simulink model "Ali_model"  (R2014b)
settings: Solver=ode4  StartTime=0.2  StopTime=11  FixedStep=0.001  RelTol=1e-3
libraries: simulink x1
settings Model: Creator=mshahria  LastModifiedBy=nlashkar

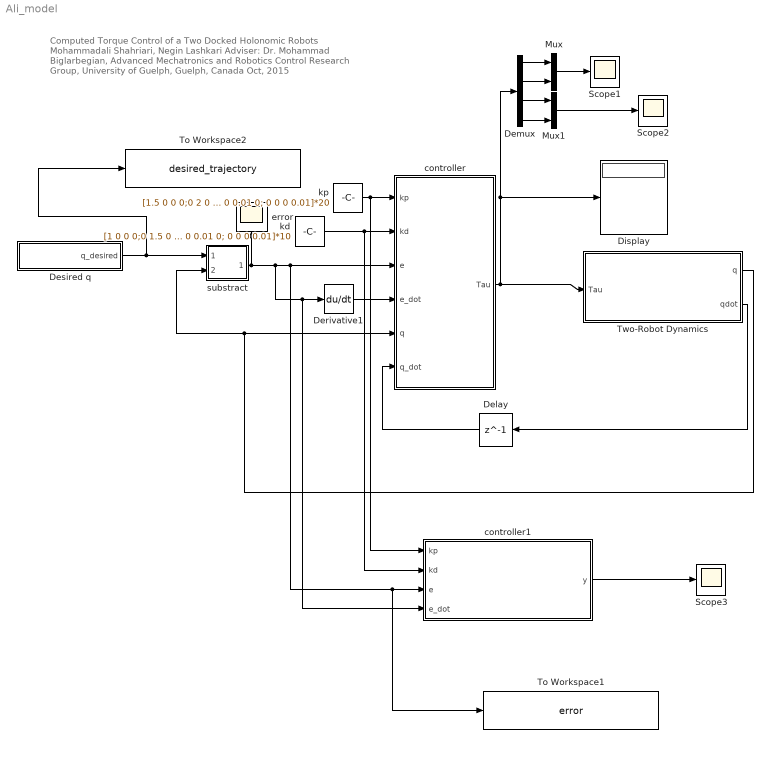
== system Ali_model ==
  note: Computed Torque Control of a Two Docked Holonomic Robots
      | Mohammadali Shahriari, Negin Lashkari
      | Adviser: Dr. Mohammad Biglarbegian,
      | Advanced Mechatronics and Robotics Control Research Group,
      |
      | University of Guelph,
      | Guelph, Canada
      |
      | Oct, 2015
  Delay : Delay  DelayLength=1  InitialCondition=zeros(8,1)
  Demux : Demux
  Derivative1 : Derivative
  "Desired q " : Subsystem
  Display : Display
  Mux : Mux  Inputs=2
  Mux1 : Mux  Inputs=2
  Scope1 : Scope
      settings: SaveName=ScopeData2
  Scope2 : Scope
      settings: SaveName=ScopeData3
  Scope3 : Scope
      settings: SaveName=ScopeData4
  To Workspace1 : ToWorkspace  VariableName=error  SampleTime=-1
  To Workspace2 : ToWorkspace  VariableName=desired_trajectory  SampleTime=-1
  Two-Robot Dynamics : Subsystem
  controller : MATLAB Function  TreatAsAtomicUnit=on
  controller1 : MATLAB Function  TreatAsAtomicUnit=on
  error : Scope
  kd : Constant  Value=[1 0 0 0;0 1.5 0 0 ; 0 0 0.01 0; 0 0 0 0.01]*10
  kp : Constant  Value=[1.5 0 0 0;0 2 0 0 ; 0 0 0.01 0; 0 0 0 0.01]*20
  substract : Subsystem
  wires:
  Two-Robot Dynamics/1(q) -> controller/5(q), substract/2(In2)
  controller/1(Tau) -> Two-Robot Dynamics/1(Tau), Display/1, Demux/1
  "Desired q "/1("q_desired ") -> To Workspace2/1, substract/1(In1)
  substract/1(Out1) -> To Workspace1/1, controller1/3(e), controller/3(e), controller1/4(e_dot), Derivative1/1, error/1
  Derivative1/1 -> controller/4(e_dot)
  kp/1 -> controller1/1(kp), controller/1(kp)
  kd/1 -> controller1/2(kd), controller/2(kd)
  Demux/1 -> Mux/1
  Demux/2 -> Mux/2
  Mux/1 -> Scope1/1
  Demux/3 -> Mux1/1
  Demux/4 -> Mux1/2
  Mux1/1 -> Scope2/1
  Two-Robot Dynamics/2(qdot) -> Delay/1
  controller1/1(y) -> Scope3/1
  Delay/1 -> controller/6(q_dot)

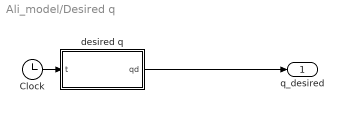
== system Ali_model/Desired q  ==
  Clock : Clock
  desired q : MATLAB Function  TreatAsAtomicUnit=on
  "q_desired " : Outport
  wires:
  Clock/1 -> desired q/1(t)
  desired q/1(qd) -> "q_desired "/1

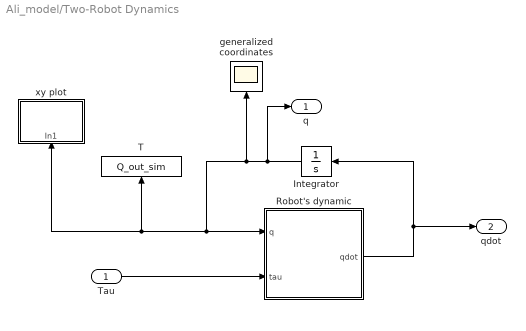
== system Ali_model/Two-Robot Dynamics ==
  Tau : Inport
  Integrator : Integrator  InitialCondition=[0.2;0.71;pi/6;pi/9;0;0;0;0]  LimitOutput=on  UpperSaturationLimit=[inf,inf,inf,inf,2,2,2,2]*0.3  LowerSaturationLimit=-[inf,inf,inf,inf,2,2,2,2]*0.3
  Robot's dynamic : MATLAB Function  TreatAsAtomicUnit=on
  T : ToWorkspace  VariableName=Q_out_sim  SampleTime=-1
  generalized coordinates : Scope
  xy plot : Subsystem
  q : Outport
  qdot : Outport  Port=2
  wires:
  Robot's dynamic/1(qdot) -> Integrator/1, qdot/1
  Integrator/1 -> q/1, Robot's dynamic/1(q), T/1, xy plot/1(In1), generalized coordinates/1
  Tau/1 -> Robot's dynamic/2(tau)

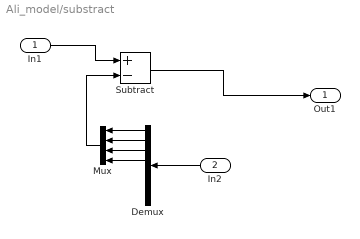
== system Ali_model/substract ==
  In1 : Inport
  In2 : Inport  Port=2
  Demux : Demux  Outputs=8
  Mux : Mux
  Subtract : Sum  Inputs=+-
  Out1 : Outport
  wires:
  Demux/2 -> Mux/2
  Mux/1 -> Subtract/2
  Demux/1 -> Mux/1
  In1/1 -> Subtract/1
  Subtract/1 -> Out1/1
  In2/1 -> Demux/1
  Demux/3 -> Mux/3
  Demux/4 -> Mux/4

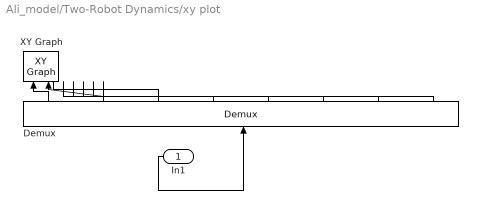
== system Ali_model/Two-Robot Dynamics/xy plot ==
  In1 : Inport
  Demux : Demux  Outputs=8
  XY Graph : simulink/Sinks/XY Graph  xmin=-3  xmax=3  ymin=-3  ymax=3  st=-1
  wires:
  Demux/1 -> XY Graph/1
  Demux/2 -> XY Graph/2
  Demux/4 -> ?
  Demux/8 -> ?
  Demux/5 -> ?
  In1/1 -> Demux/1
  Demux/3 -> ?
  Demux/7 -> ?
  Demux/6 -> ?

== matlab function Ali_model/controller ==
  data: kp input; kd input; e input; e_dot input; q input; Tau output; q_dot input
function Tau= fcn(kp,kd,e,e_dot,q,q_dot)

theta_1= q(3);
theta_2= q(4);

theta_dot1=q(7);
theta_dot2=q(8);

x_dotdot=q_dot(5);
y_dotdot=q_dot(6);
theta_dotdot1=q_dot(7);
theta_dotdot2=q_dot(8);

% to avoid singularity on the docked mechanism:

% if abs(theta_1-theta_2)<1e-2
%     if theta_dot2>=0
%      theta_2=theta_1+0.0001;
%     else
%      theta_2=theta_1-0.0001;
%     end
% end

%---------------------------------------------

Tau=Tau_computed(theta_1,theta_2,theta_dot1,theta_dot2,theta_dotdot1,theta_dotdot2,x_dotdot,y_dotdot);
Tau=Tau+B_inverse(theta_1,theta_2)*(kp*e+kd*e_dot);

== matlab function Ali_model/Desired q /desired q ==
  data: t input; qd output
function qd= fcn(t)
% if t<=10
qd=q_desired(t);
% else
%  qd=q_desired(10);
% end

== matlab function Ali_model/Two-Robot Dynamics/Robot's dynamic ==
  data: q input; qdot output; tau input
function qdot= fcn(q,tau)


qdot=zeros(8,1);



% input torque:

tau_l1=tau(1);
tau_r1=tau(2);
tau_l2=tau(3);
tau_r2=tau(4);

% defining ode: 

theta_1= q(3);
theta_2= q(4);
theta_dot1=q(7);
theta_dot2=q(8);



qdoubledot=Qdotdot(tau_l1,tau_l2,tau_r1,tau_r2,theta_1,theta_2,theta_dot1,theta_dot2);



qdot(1)=q(5);
qdot(2)=q(6);
qdot(3)=q(7);
qdot(4)=q(8);
qdot(5)=qdoubledot(1);
qdot(6)=qdoubledot(2);
qdot(7)=qdoubledot(3);
qdot(8)=qdoubledot(4);

end

== matlab function Ali_model/controller1 ==
  data: kp input; kd input; e input; e_dot input; y output
function y= fcn(kp,kd,e,e_dot)

y=kp*e+kd*e_dot;
